simulink model "test1_1"  (R2018b)
settings: Solver=FixedStepAuto  StartTime=0.0  StopTime=0.2  FixedStep=1e-6  RelTol=1e-3
libraries: dsparch4 x3, dspstat3 x2, dspmathops x2, commchan3 x1
settings Model: Creator=Aurora  LastModifiedBy=Aurora

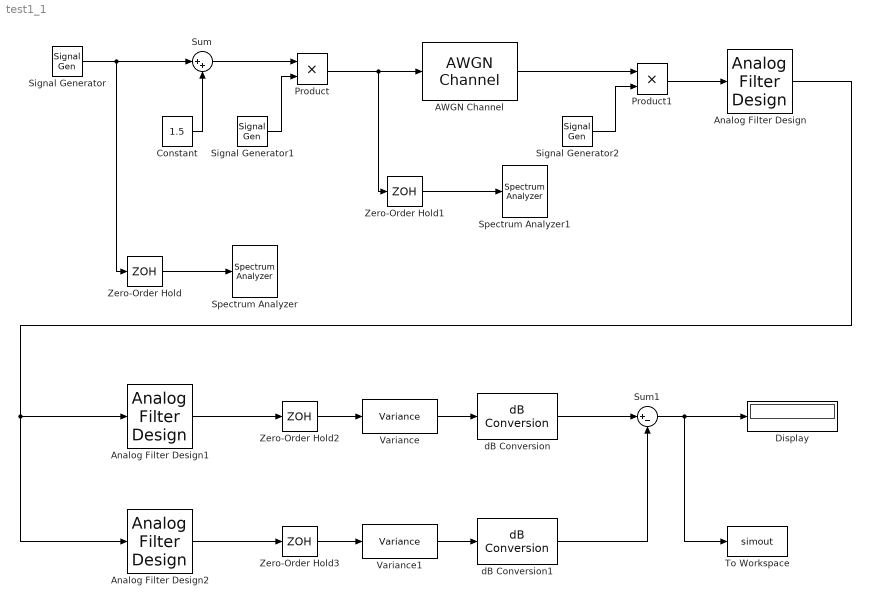
== system test1_1 ==
  AWGN Channel : commchan3/AWGN Channel  InputProcessing=Columns as channels (frame based)  seed=67  noiseMode="Signal to noise ratio  (SNR)"  EbNodB=10  EsNodB=10  SNRdB=10  bitsPerSym=1  Ps=1  Tsym=1  variance=1
  Analog Filter Design : dsparch4/Analog Filter Design  method=Butterworth  filttype=Lowpass  N=8  Wlo=2*pi*3000  Whi=80  Rp=2  Rs=40
  Analog Filter Design1 : dsparch4/Analog Filter Design  method=Butterworth  filttype=Bandpass  N=1  Wlo=2*pi*2800  Whi=2*pi*3200  Rp=2  Rs=40
  Analog Filter Design2 : dsparch4/Analog Filter Design  method=Butterworth  filttype=Bandstop  N=8  Wlo=2*pi*2800  Whi=2*pi*3200  Rp=2  Rs=40
  Constant : Constant  Value=1.5
  Display : Display
  Product : Product
  Product1 : Product
  Signal Generator : SignalGenerator  Frequency=3000
  Signal Generator1 : SignalGenerator  Frequency=90000
  Signal Generator2 : SignalGenerator  Frequency=90000
  Spectrum Analyzer : SpectrumAnalyzer
  Spectrum Analyzer1 : SpectrumAnalyzer
  Sum : Sum  Inputs=|++
  Sum1 : Sum  Inputs=|+-
  To Workspace : ToWorkspace  VariableName=simout  SaveFormat=Timeseries  SampleTime=-1
  Variance : dspstat3/Variance  run=on  InputProcessing=Columns as channels (frame based)  reset_popup=None  directionMode=Each column  dimension=1  roiEnable=off  roiType=Rectangles  roiPortion=Entire ROI  roiOutput=Individual statistics for each ROI  roiFlag=off  roundingMode=Floor  overflowMode=off
      settings: SourceProductName=DSP System Toolbox
  Variance1 : dspstat3/Variance  run=on  InputProcessing=Columns as channels (frame based)  reset_popup=None  directionMode=Each column  dimension=1  roiEnable=off  roiType=Rectangles  roiPortion=Entire ROI  roiOutput=Individual statistics for each ROI  roiFlag=off  roundingMode=Floor  overflowMode=off
      settings: SourceProductName=DSP System Toolbox
  Zero-Order Hold{,1..3} (4 alike) : ZeroOrderHold  SampleTime=-1
  dB Conversion : dspmathops/dB Conversion  dBtype=dB  intype=Power  R=1  fuzz=on
      settings: SourceProductName=DSP System Toolbox
  dB Conversion1 : dspmathops/dB Conversion  dBtype=dB  intype=Power  R=1  fuzz=on
      settings: SourceProductName=DSP System Toolbox
  wires:
  Signal Generator/1 -> Zero-Order Hold/1, Sum/1
  Sum/1 -> Product/1
  Constant/1 -> Sum/2
  Signal Generator1/1 -> Product/2
  Product/1 -> Zero-Order Hold1/1, AWGN Channel/1
  AWGN Channel/1 -> Product1/1
  Signal Generator2/1 -> Product1/2
  Product1/1 -> Analog Filter Design/1
  Zero-Order Hold1/1 -> Spectrum Analyzer1/1
  Zero-Order Hold/1 -> Spectrum Analyzer/1
  Variance/1 -> dB Conversion/1
  Analog Filter Design1/1 -> Zero-Order Hold2/1
  Zero-Order Hold2/1 -> Variance/1
  Analog Filter Design2/1 -> Zero-Order Hold3/1
  Zero-Order Hold3/1 -> Variance1/1
  Variance1/1 -> dB Conversion1/1
  Sum1/1 -> Display/1, To Workspace/1
  dB Conversion/1 -> Sum1/1
  dB Conversion1/1 -> Sum1/2
  Analog Filter Design/1 -> Analog Filter Design2/1, Analog Filter Design1/1
